simulink model "simulacionPI_Discreto"  (R2022b)
settings: Solver=VariableStepAuto  StartTime=0.0  StopTime=1  RelTol=1e-3
values from neighbouring files (symbols this model uses):
  den = [L*J, L*b + R*J, R*b + Kt*Km]    [parametrosMotorDC.m]
  num = [Kt]    [parametrosMotorDC.m]
  Ts = 0.001    [comportamientoMotorConPID.m]
undefined symbols (not defined in the file or in its folder): den_z, num_z
settings Model: Creator=hp  LastModifiedBy=hp

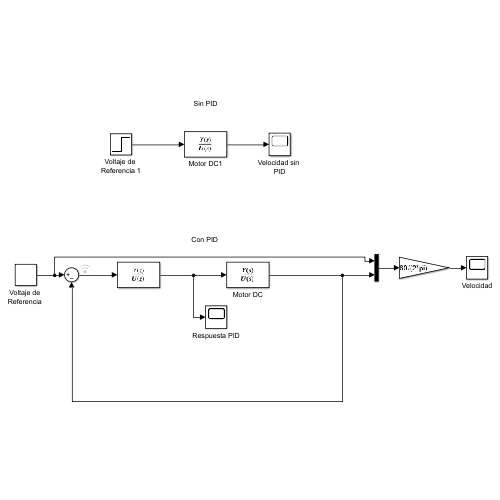
[thumbnail: Simulink's stored preview of the top-level diagram]
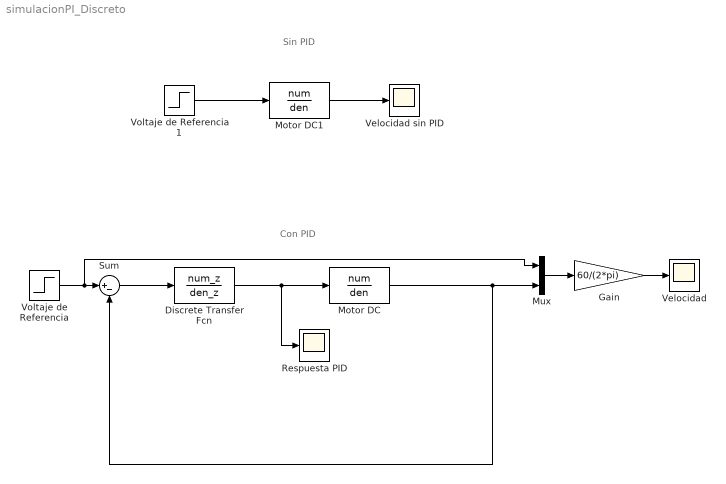
== system simulacionPI_Discreto ==
  note: Con PID
  note: Sin PID
  Discrete Transfer Fcn : DiscreteTransferFcn  Numerator=num_z  Denominator=den_z  SampleTime=Ts
  Gain : Gain  Gain=60/(2*pi)
  Motor DC : TransferFcn  Numerator=num  Denominator=den
  Motor DC1 : TransferFcn  Numerator=num  Denominator=den
  Mux : Mux  Inputs=2
  Respuesta PID : Scope
  Sum : Sum  Inputs=|+-
  Velocidad : Scope
  Velocidad sin PID : Scope
  "Voltaje de Referencia " : Step  Time=0.1  After=1500*2*pi/60  SampleTime=Ts
  Voltaje de Referencia 1 : Step  Time=0.1  After=6  SampleTime=0
  wires:
  Voltaje de Referencia 1/1 -> Motor DC1/1
  Discrete Transfer Fcn/1 -> Respuesta PID/1, Motor DC/1
  Motor DC/1 -> Mux/2, Sum/2
  Sum/1 -> Discrete Transfer Fcn/1
  Motor DC1/1 -> Velocidad sin PID/1
  "Voltaje de Referencia "/1 -> Mux/1, Sum/1
  Gain/1 -> Velocidad/1
  Mux/1 -> Gain/1
